simulink model "Group69_Simulink"  (R2021b)
settings: Solver=ode45  StartTime=0.0  StopTime=T  RelTol=1e-12
values from neighbouring files (symbols this model uses):
  A_BN_0 = A_NB_0'    [Group69_Matlab.m]
  m = [0.01 0.05 0.01]'    [Group69_Matlab.m]
  R3H0 = orbit.Re^3*H0    [Group69_Matlab.m]
  w0 = [wx0,wy0,wz0]'    [Group69_Matlab.m]
undefined symbols (not defined in the file or in its folder): gyro, hs, inertia, mag, orbit, r0, rw, sc, t, v0
libraries: matrix_library x8, simulink_extras x6
settings Model: Creator=rocco_larocca  LastModifiedBy=rocco_larocca

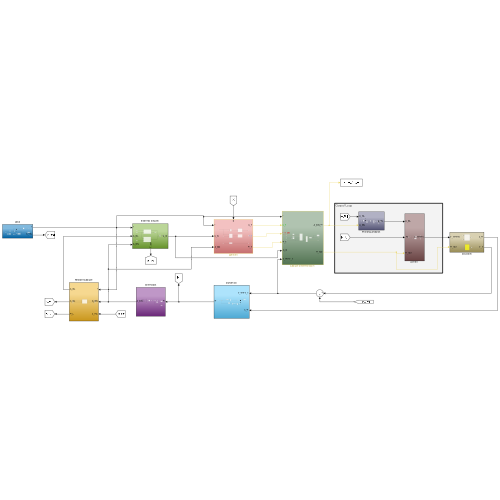
[thumbnail: Simulink's stored preview of the top-level diagram]
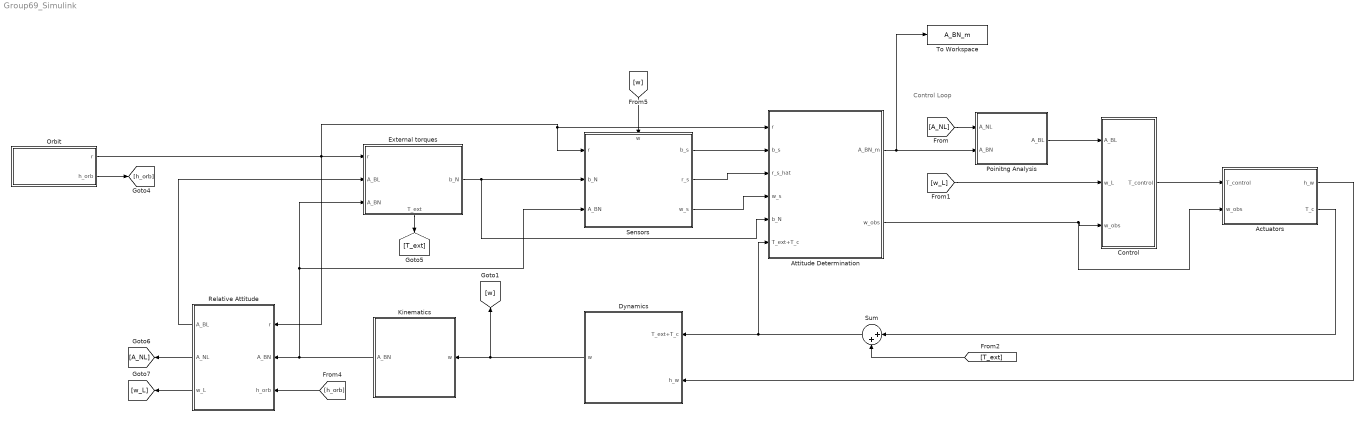
== system Group69_Simulink ==
  note: Control Loop
  Actuators : Subsystem
  "Attitude Determination " : Subsystem
  Control : Subsystem
  Dynamics : Subsystem
  External torques : Subsystem
      settings: PortSchema="{\"entries\":[{\"content\":{\"sides\":[{\"content\":{\"connectorIds\":[\"In1\",\"In2\",\"In3\"]},\"type\":\"ConnectorPlacement.EquallySpacedRectSide\",\"uuid\":\"c5dd5657-11cd-46fc-a813-74747ea81146\"},{\"content\":{\"connectorIds\":[\"Out1\"],\"side\":\"RIGHT\"},\"type\":\"ConnectorPlacement.EquallySpacedRectSide\",\"uuid\":\"ce8cbc86-0401-4f30-83b3-f262a6771dee\"},{\"content\":{\"connectorIds\":[],\"side\":\"TOP\"},\"type\":\"ConnectorPlacement.EquallySpacedRectSide\",\"uuid\":\"54f7f4d9-1155-478d-825b-4623d6763012\"},{\"content\":{\"connectorIds\":[\"Out2\"],\"side\":\"BOTTOM\"},\"type\":\"ConnectorPlacement.EquallySpacedRectSide\",\"uuid\":\"9bbeb954-f49a-41a5-9c63-5058200ec5df\"}]},\"type\":\"ConnectorPlacement.EquallySpacedConnector\",\"uuid\":\"ae160f86-5b24-4f86-a6f1-a9e1b48113ae\"}],\"packageUris\":[\"http://schema.mathworks.com/mf0/Connector/R2020b\"],\"version\":\"1.0\"}"
  Kinematics : Subsystem
  Orbit : Subsystem
  Poinitng Analysis : Subsystem
  Relative Attitude : Subsystem
  Sensors : Subsystem
      settings: PortSchema="{\"entries\":[{\"content\":{\"sides\":[{\"content\":{\"connectorIds\":[\"In1\",\"In2\",\"In3\"]},\"type\":\"ConnectorPlacement.EquallySpacedRectSide\",\"uuid\":\"26d18e7d-7ebd-44fe-966b-e5460611b065\"},{\"content\":{\"connectorIds\":[\"Out1\",\"Out2\",\"Out3\"],\"side\":\"RIGHT\"},\"type\":\"ConnectorPlacement.EquallySpacedRectSide\",\"uuid\":\"31c3f243-0c2a-44fb-92ca-61b97f920180\"},{\"content\":{\"connectorIds\":[\"In4\"],\"side\":\"TOP\"},\"type\":\"ConnectorPlacement.EquallySpacedRectSide\",\"uuid\":\"517f47c7-f5cc-49ce-9a5d-236df56a8d72\"}]},\"type\":\"ConnectorPlacement.EquallySpacedConnector\",\"uuid\":\"aa3704da-9102-4b45-8547-3c2cdec151e6\"}],\"packageUris\":[\"http://schema.mathworks.com/mf0/Connector/R2020b\"],\"version\":\"1.0\"}"
  Sum : Sum  Inputs=|++
  To Workspace : ToWorkspace  VariableName=A_BN_m  SaveFormat=Timeseries  SampleTime=-1
  wires:
  Dynamics/1(w) -> [w], Kinematics/1(w)
  Kinematics/1(A_BN) -> Sensors/3(A_BN), External torques/3(A_BN), Relative Attitude/2(A_BN)
  [h_orb] -> Relative Attitude/3(h_orb)
  Orbit/1(r) -> Relative Attitude/1(r), Sensors/1(r), "Attitude Determination "/1(r), External torques/1(r)
  Orbit/2(h_orb) -> [h_orb]
  Relative Attitude/1(A_BL) -> External torques/2(A_BL)
  External torques/2(T_ext) -> [T_ext]
  External torques/1(b_N) -> "Attitude Determination "/5(" b_N "), Sensors/2(b_N)
  [w] -> Sensors/4(w)
  Sensors/2(r_s) -> "Attitude Determination "/3(r_s_hat)
  Sensors/1(b_s) -> "Attitude Determination "/2(b_s)
  Sensors/3(w_s) -> "Attitude Determination "/4(w_s)
  Relative Attitude/2(A_NL) -> [A_NL]
  Relative Attitude/3(w_L) -> [w_L]
  [T_ext] -> Sum/2
  Actuators/2(T_c) -> Sum/1
  Sum/1 -> "Attitude Determination "/6(T_ext+T_c), Dynamics/1(T_ext+T_c)
  Actuators/1(h_w) -> Dynamics/2(h_w)
  [A_NL] -> Poinitng Analysis/1(A_NL)
  "Attitude Determination "/1(A_BN_m) -> To Workspace/1, Poinitng Analysis/2(A_BN)
  Poinitng Analysis/1(A_BL) -> Control/1(A_BL)
  "Attitude Determination "/2(w_obs) -> Actuators/2(w_obs), Control/3("w_obs ")
  Control/1(T_control) -> Actuators/1(T_control)
  [w_L] -> Control/2(" w_L ")

== system Group69_Simulink/Actuators ==
  T_control : Inport
  w_obs : Inport  Port=2
  Inertia Wheel : Subsystem
      settings: PortSchema="{\"entries\":[{\"content\":{\"sides\":[{\"content\":{\"connectorIds\":[]},\"type\":\"ConnectorPlacement.EquallySpacedRectSide\",\"uuid\":\"666c479f-9627-4b2d-b95f-c868510cc6c0\"},{\"content\":{\"connectorIds\":[],\"side\":\"RIGHT\"},\"type\":\"ConnectorPlacement.EquallySpacedRectSide\",\"uuid\":\"1c954fcd-03c3-4322-8621-3bafaef6b025\"},{\"content\":{\"connectorIds\":[],\"side\":\"TOP\"},\"type\":\"ConnectorPlacement.EquallySpacedRectSide\",\"uuid\":\"948c880d-c243-4d30-bb3c-bd369bf7890c\"},{\"content\":{\"connectorIds\":[\"Out1\"],\"side\":\"BOTTOM\"},\"type\":\"ConnectorPlacement.EquallySpacedRectSide\",\"uuid\":\"e6b921d4-3671-426f-8404-dd4d7604816b\"}]},\"type\":\"ConnectorPlacement.EquallySpacedConnector\",\"uuid\":\"4740817b-bbe6-45b7-9db2-684bb8b90ddd\"}],\"packageUris\":[\"http://schema.mathworks.com/mf0/Connector/R2020b\"],\"version\":\"1.0\"}"
  Reaction Wheels : Subsystem
  h_w : Outport
  T_c : Outport  Port=2
  wires:
  T_control/1 -> Reaction Wheels/1(T_control)
  Reaction Wheels/1(T_c) -> T_c/1
  w_obs/1 -> Reaction Wheels/2(w_obs)
  Inertia Wheel/1(h_w) -> h_w/1

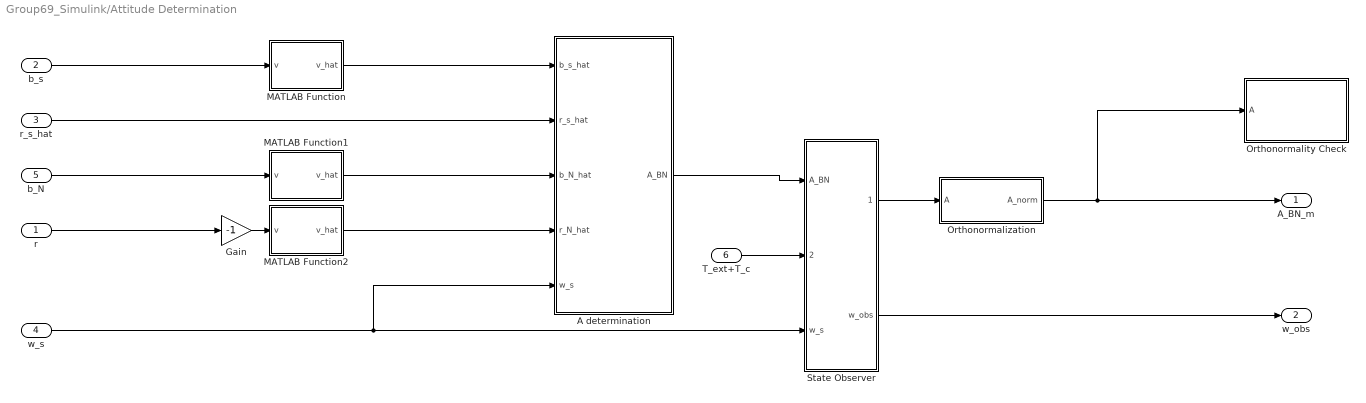
== system Group69_Simulink/Attitude Determination  ==
  r : Inport
  b_s : Inport  Port=2
  r_s_hat : Inport  Port=3
  w_s : Inport  Port=4
  " b_N " : Inport  Port=5
  T_ext+T_c : Inport  Port=6
  A determination : Subsystem
  Gain : Gain  Gain=-1
  MATLAB Function : MATLAB Function  TreatAsAtomicUnit=on
  MATLAB Function1 : MATLAB Function  TreatAsAtomicUnit=on
  MATLAB Function2 : MATLAB Function  TreatAsAtomicUnit=on
  Orthonormality Check : Subsystem
  Orthonormalization : Subsystem
  State Observer : Subsystem
  A_BN_m : Outport
  w_obs : Outport  Port=2
  wires:
  r/1 -> Gain/1
  b_s/1 -> MATLAB Function/1(v)
  Gain/1 -> MATLAB Function2/1(v)
  " b_N "/1 -> MATLAB Function1/1(v)
  r_s_hat/1 -> A determination/2(r_s_hat)
  Orthonormalization/1(A_norm) -> Orthonormality Check/1(A), A_BN_m/1
  w_s/1 -> State Observer/3(w_s), A determination/5(w_s)
  State Observer/1(A_BN_obs) -> Orthonormalization/1(A)
  A determination/1(A_BN) -> State Observer/1(A_BN)
  MATLAB Function/1(v_hat) -> A determination/1(b_s_hat)
  MATLAB Function1/1(v_hat) -> A determination/3(b_N_hat)
  MATLAB Function2/1(v_hat) -> A determination/4(r_N_hat)
  T_ext+T_c/1 -> State Observer/2(T_ext+T_c)
  State Observer/2(w_obs) -> w_obs/1

== system Group69_Simulink/Control ==
  A_BL : Inport
  " w_L " : Inport  Port=2
  "w_obs " : Inport  Port=3
  Clock : Clock
  Detumbling : Subsystem  TreatAsAtomicUnit=on
  If Action Subsystem : Subsystem  TreatAsAtomicUnit=on
  Merge : Merge
  Phase Identification : If  IfExpression=u1<(300)
  T_control : Outport
  wires:
  Phase Identification/2 -> If Action Subsystem/Action
  A_BL/1 -> If Action Subsystem/1(A_BL)
  " w_L "/1 -> If Action Subsystem/2("w_L  ")
  Clock/1 -> Phase Identification/1
  "w_obs "/1 -> Detumbling/1(w_obs), If Action Subsystem/3(w_b)
  Merge/1 -> T_control/1
  Phase Identification/1 -> Detumbling/Action
  Detumbling/1(T_id) -> Merge/1
  If Action Subsystem/1(T_id) -> Merge/2

== system Group69_Simulink/Dynamics ==
  note: adding inertia wheel
  T_ext+T_c : Inport
  h_w : Inport  Port=2
  Cross Product : matrix_library/Cross Product
      settings: SourceProductBaseCode=SL
  Product : Product  Multiplication=Matrix(*)
  Product1 : Product  Multiplication=Matrix(*)
  Sum : Sum  Inputs=+-
  Sum1 : Sum
  inp1 : Constant  Value=sc.I_inv
  inp2 : Constant  Value=sc.I
  int1 : Integrator  InitialCondition=w0
  out1 : ToWorkspace  VariableName=w  SaveFormat=Timeseries  SampleTime=-1
  w : Outport
  wires:
  Sum/1 -> Product1/2
  Product1/1 -> int1/1
  Product/1 -> Sum1/2
  int1/1 -> Cross Product/1, Product/2, out1/1, w/1
  inp1/1 -> Product1/1
  T_ext+T_c/1 -> Sum/1
  inp2/1 -> Product/1
  Sum1/1 -> Cross Product/2
  h_w/1 -> Sum1/1
  Cross Product/1 -> Sum/2

== system Group69_Simulink/External torques ==
  r : Inport
  A_BL : Inport  Port=2
  A_BN : Inport  Port=3
  Gravity Gradient Torque : Subsystem
  Magnetic Torque : Subsystem
  Sum : Sum
  b_N : Outport
  T_ext : Outport  Port=2
  wires:
  A_BL/1 -> Gravity Gradient Torque/2(A_BL)
  r/1 -> Gravity Gradient Torque/1(r), Magnetic Torque/2(r)
  A_BN/1 -> Magnetic Torque/1(A_BN)
  Sum/1 -> T_ext/1
  Magnetic Torque/1(T_magnetic) -> Sum/1
  Magnetic Torque/2(b_N) -> b_N/1
  Gravity Gradient Torque/1(T_gravity) -> Sum/2

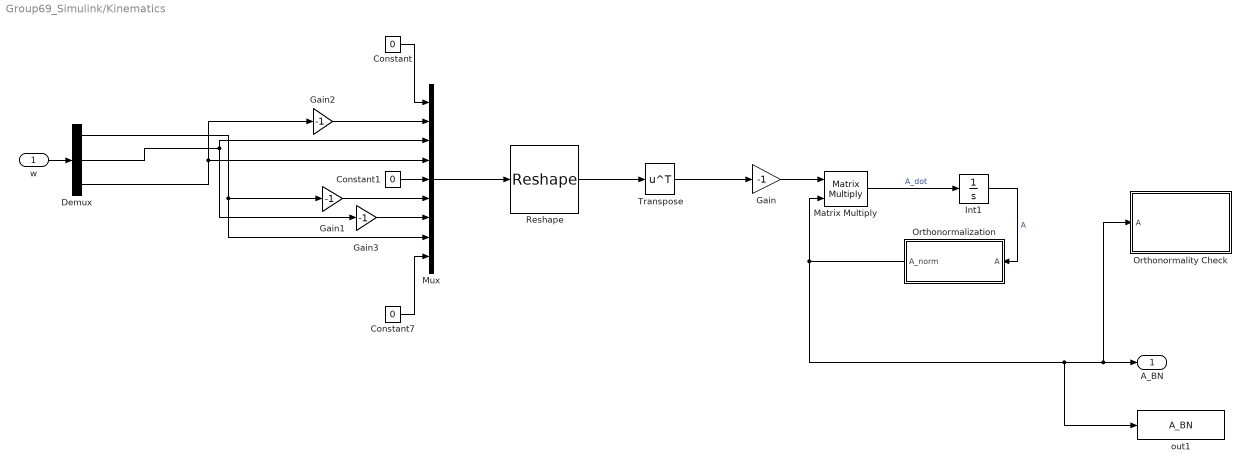
== system Group69_Simulink/Kinematics ==
  w : Inport
  Constant : Constant  Value=0
  Constant1 : Constant  Value=0
  Constant7 : Constant  Value=0
  Demux : Demux  Outputs=3
  Gain{,1..3} (4 alike) : Gain  Gain=-1
  Int1 : Integrator  InitialCondition=A_BN_0
  Matrix Multiply : Product  Multiplication=Matrix(*)
  Mux : Mux  Inputs=9
  Orthonormality Check : Subsystem
  Orthonormalization : Subsystem
  Reshape : Reshape  OutputDimensionality=Customize  OutputDimensions=[3,3]
  Transpose : Math  Operator=transpose  SaturateOnIntegerOverflow=on
  out1 : ToWorkspace  VariableName=A_BN  SaveFormat=Timeseries  SampleTime=-1
  A_BN : Outport
  wires:
  Matrix Multiply/1 -> Int1/1  "A_dot"
  Gain/1 -> Matrix Multiply/1
  Int1/1 -> Orthonormalization/1(A)  "A"
  Orthonormalization/1(A_norm) -> Orthonormality Check/1(A), A_BN/1, out1/1, Matrix Multiply/2
  Constant1/1 -> Mux/5
  Constant/1 -> Mux/1
  Gain1/1 -> Mux/6
  Mux/1 -> Reshape/1
  Gain2/1 -> Mux/2
  Gain3/1 -> Mux/7
  Demux/1 -> Mux/8, Gain1/1
  Constant7/1 -> Mux/9
  w/1 -> Demux/1
  Reshape/1 -> Transpose/1
  Demux/3 -> Mux/4, Gain2/1
  Demux/2 -> Mux/3, Gain3/1
  Transpose/1 -> Gain/1

== system Group69_Simulink/Orbit ==
  Constant : Constant  Value=-3
  Cross Product : matrix_library/Cross Product
      settings: SourceProductBaseCode=SL
  Gain : Gain  Gain=orbit.mu
  Gain1 : Gain  Gain=-1
  MATLAB Function : MATLAB Function  TreatAsAtomicUnit=on
  MatrixMultiply : Product
  Power : Math  Operator=pow  SaturateOnIntegerOverflow=on
  Terminator : Terminator
  To Workspace3 : ToWorkspace  VariableName=r  SaveFormat=Timeseries  SampleTime=-1
  int1 : Integrator  InitialCondition=v0
  int2 : Integrator  InitialCondition=r0
  r : Outport
  h_orb : Outport  Port=2
  wires:
  Gain/1 -> Gain1/1
  int2/1 -> MATLAB Function/1(v), To Workspace3/1, Cross Product/1, r/1, MatrixMultiply/1
  Gain1/1 -> int1/1
  int1/1 -> Cross Product/2, int2/1
  MatrixMultiply/1 -> Gain/1
  Power/1 -> MatrixMultiply/2
  Constant/1 -> Power/2
  Cross Product/1 -> h_orb/1
  MATLAB Function/2(norm_v) -> Power/1
  MATLAB Function/1(v_hat) -> Terminator/1

== system Group69_Simulink/Poinitng Analysis ==
  A_NL : Inport
  A_BN : Inport  Port=2
  Acos : Trigonometry  Operator=acos
  Dot Product : DotProduct  InputSameDT=on  OutDataTypeStr=Inherit: Inherit via internal rule
  MatrixMultiply : Product  Multiplication=Matrix(*)
  MatrixMultiply1 : Product  Multiplication=Matrix(*)
  Nadir Pointing in Body : Constant  Value=[ 1 0 0 ]
  Nadir Pointing in LVLH : Constant  Value=[ 1 0 0 ]
  Radians to Degrees : simulink_extras/Transformations/Radians to Degrees
  Scope : Scope
  To Workspace : ToWorkspace  VariableName=ang_err  SaveFormat=Timeseries  SampleTime=-1
  A_BL : Outport
  wires:
  A_NL/1 -> MatrixMultiply/2
  A_BN/1 -> MatrixMultiply/1
  MatrixMultiply/1 -> MatrixMultiply1/1, A_BL/1
  Nadir Pointing in LVLH/1 -> MatrixMultiply1/2
  MatrixMultiply1/1 -> Dot Product/1
  Nadir Pointing in Body/1 -> Dot Product/2
  Dot Product/1 -> Acos/1
  Acos/1 -> Radians to Degrees/1
  Radians to Degrees/1 -> To Workspace/1, Scope/1

== system Group69_Simulink/Relative Attitude ==
  r : Inport
  A_BN : Inport  Port=2
  h_orb : Inport  Port=3
  moving to LVLH and inertial : Subsystem
  A_BL : Outport
  A_NL : Outport  Port=2
  w_L : Outport  Port=3
  wires:
  h_orb/1 -> moving to LVLH and inertial/3(h_orb)
  moving to LVLH and inertial/1(A_BL) -> A_BL/1
  moving to LVLH and inertial/2(A_NL) -> A_NL/1
  A_BN/1 -> moving to LVLH and inertial/1(A_BN)
  r/1 -> moving to LVLH and inertial/2(r)
  moving to LVLH and inertial/3(w_L) -> w_L/1

== system Group69_Simulink/Sensors ==
  r : Inport
  b_N : Inport  Port=2
  A_BN : Inport  Port=3
  w : Inport  Port=4
  Earth Horizon Sensor : Subsystem
  Field of view check and r to body : Subsystem
  From inertial to body : Product  Multiplication=Matrix(*)
  Gyroscope : Subsystem
  Magnetic Sensor : Subsystem
  b_s : Outport
  r_s : Outport  Port=2
  w_s : Outport  Port=3
  wires:
  A_BN/1 -> Field of view check and r to body/1(A_BN), From inertial to body/1
  r/1 -> Field of view check and r to body/2(r)
  Magnetic Sensor/1(b_S) -> b_s/1
  b_N/1 -> From inertial to body/2
  From inertial to body/1 -> Magnetic Sensor/1(b_B)
  Earth Horizon Sensor/1(r_s) -> r_s/1
  Field of view check and r to body/1(r_B) -> Earth Horizon Sensor/1(r_B)
  w/1 -> Gyroscope/1(w)
  Gyroscope/1(w_s) -> w_s/1

== system Group69_Simulink/Actuators/Inertia Wheel ==
  Clock1 : Clock
  Gain : Gain  Gain=0
  MatrixMultiply : Product  Multiplication=Matrix(*)
  Scope : Scope
  Switch : Switch  Criteria=u2 > Threshold  Threshold=t.detumbling
  inp1 : Constant  Value=inertia.I
  inp2 : Constant  Value=inertia.w
  h_w : Outport
  wires:
  inp1/1 -> MatrixMultiply/1
  Gain/1 -> Switch/3
  Clock1/1 -> Switch/2
  inp2/1 -> MatrixMultiply/2
  MatrixMultiply/1 -> Gain/1, Switch/1
  Switch/1 -> h_w/1, Scope/1

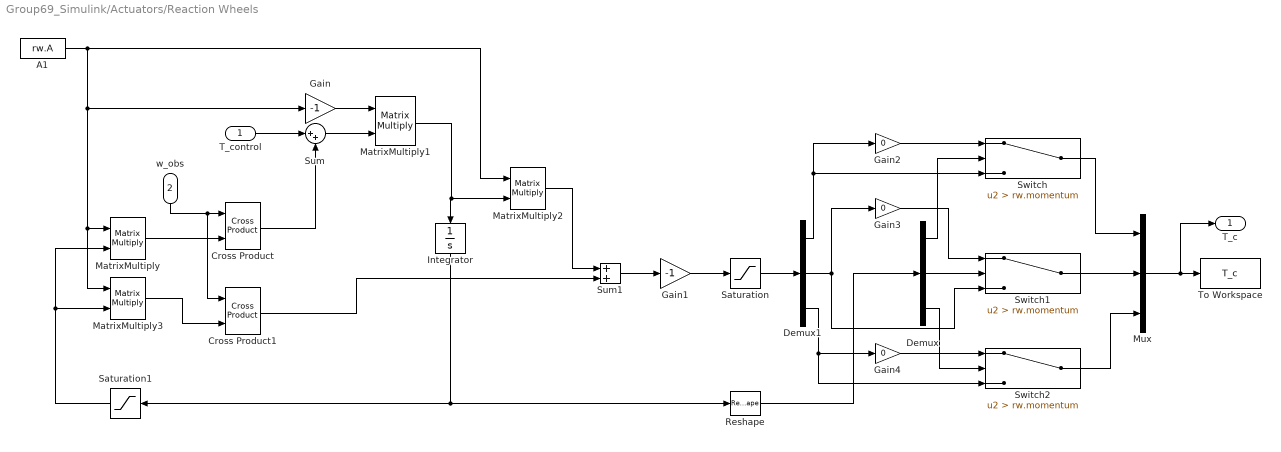
== system Group69_Simulink/Actuators/Reaction Wheels ==
  T_control : Inport
  w_obs : Inport  Port=2
  A1 : Constant  Value=rw.A
  Cross Product : matrix_library/Cross Product
      settings: SourceProductBaseCode=SL
  Cross Product1 : matrix_library/Cross Product
      settings: SourceProductBaseCode=SL
  Demux : Demux  Outputs=3
  Demux1 : Demux  Outputs=3
  Gain : Gain  Gain=-1
  Gain1 : Gain  Gain=-1
  Gain2 : Gain  Gain=0
  Gain3 : Gain  Gain=0
  Gain4 : Gain  Gain=0
  Integrator : Integrator
  MatrixMultiply{,1..3} (4 alike) : Product  Multiplication=Matrix(*)
  Mux : Mux  Inputs=3
  Reshape : Reshape  OutputDimensionality=Column vector (2-D)
  Saturation : Saturate  UpperLimit=rw.maxtorque  LowerLimit=-rw.maxtorque  LinearizeAsGain=off
  Saturation1 : Saturate  UpperLimit=rw.momentum  LowerLimit=-rw.momentum
  Sum : Sum  Inputs=|++
  Sum1 : Sum
  Switch : Switch  Criteria=u2 > Threshold  Threshold=rw.momentum
  Switch1 : Switch  Criteria=u2 > Threshold  Threshold=rw.momentum
  Switch2 : Switch  Criteria=u2 > Threshold  Threshold=rw.momentum
  To Workspace : ToWorkspace  VariableName=T_c  SaveFormat=Timeseries  SampleTime=-1
  T_c : Outport
  wires:
  w_obs/1 -> Cross Product1/1, Cross Product/1
  MatrixMultiply1/1 -> Integrator/1, MatrixMultiply2/2
  Saturation1/1 -> MatrixMultiply/2, MatrixMultiply3/2
  Demux1/1 -> Switch/3, Gain2/1
  Demux1/2 -> Switch1/3, Gain3/1
  Mux/1 -> To Workspace/1, T_c/1
  MatrixMultiply/1 -> Cross Product/2
  T_control/1 -> Sum/1
  Cross Product1/1 -> Sum1/2
  Cross Product/1 -> Sum/2
  Sum/1 -> MatrixMultiply1/2
  Gain/1 -> MatrixMultiply1/1
  MatrixMultiply2/1 -> Sum1/1
  Sum1/1 -> Gain1/1
  Gain1/1 -> Saturation/1
  MatrixMultiply3/1 -> Cross Product1/2
  Demux/2 -> Switch1/2
  Demux/3 -> Switch2/2
  Switch1/1 -> Mux/2
  Gain3/1 -> Switch1/1
  Gain2/1 -> Switch/1
  Switch/1 -> Mux/1
  Demux/1 -> Switch/2
  Gain4/1 -> Switch2/1
  Switch2/1 -> Mux/3
  Reshape/1 -> Demux/1
  Saturation/1 -> Demux1/1
  Demux1/3 -> Switch2/3, Gain4/1
  Integrator/1 -> Saturation1/1, Reshape/1
  A1/1 -> MatrixMultiply2/1, Gain/1, MatrixMultiply3/1, MatrixMultiply/1

== system Group69_Simulink/Attitude Determination /A determination ==
  b_s_hat : Inport
  r_s_hat : Inport  Port=2
  b_N_hat : Inport  Port=3
  r_N_hat : Inport  Port=4
  w_s : Inport  Port=5
  A_det : MATLAB Function  TreatAsAtomicUnit=on
  Reshape{,2..3,5} (4 alike) : Reshape  OutputDimensionality=Column vector (2-D)
  Subsystem : Subsystem
  A_BN : Outport
  wires:
  b_s_hat/1 -> Reshape/1
  r_s_hat/1 -> Reshape2/1
  b_N_hat/1 -> Reshape3/1
  r_N_hat/1 -> Reshape5/1
  Reshape/1 -> A_det/1(b_s_hat)
  Reshape2/1 -> A_det/2(r_s_hat)
  Reshape3/1 -> A_det/3(b_N_hat)
  Reshape5/1 -> A_det/4(r_N_hat)
  w_s/1 -> A_det/5(wb_sens)
  Subsystem/1(A_BN) -> A_BN/1
  Subsystem/2(A_prev) -> A_det/6(A_prev)
  A_det/2(c) -> Subsystem/2(c)
  A_det/1(A) -> Subsystem/1(A)
  A_det/3(A_dot) -> Subsystem/3(A_dot)

== system Group69_Simulink/Attitude Determination /Orthonormality Check ==
  A : Inport
  Determinant : Subsystem  Commented=on
  MATLAB Function : MATLAB Function  TreatAsAtomicUnit=on
  Scope : Scope
  wires:
  A/1 -> MATLAB Function/1(A)
  MATLAB Function/1(detA) -> Scope/1

== system Group69_Simulink/Attitude Determination /Orthonormalization ==
  A : Inport
  Gain : Gain  Gain=1.5
  Gain1 : Gain  Gain=0.5
  Matrix Multiply : Product  Multiplication=Matrix(*)
  Matrix Multiply1 : Product  Multiplication=Matrix(*)
  Sum : Sum  Inputs=+-
  Transpose : Math  Operator=transpose  SaturateOnIntegerOverflow=on
  A_norm : Outport
  wires:
  Gain/1 -> Sum/1
  Transpose/1 -> Matrix Multiply/2
  A/1 -> Transpose/1, Gain1/1, Matrix Multiply/1, Gain/1
  Matrix Multiply1/1 -> Sum/2
  Sum/1 -> A_norm/1
  Matrix Multiply/1 -> Matrix Multiply1/1
  Gain1/1 -> Matrix Multiply1/2

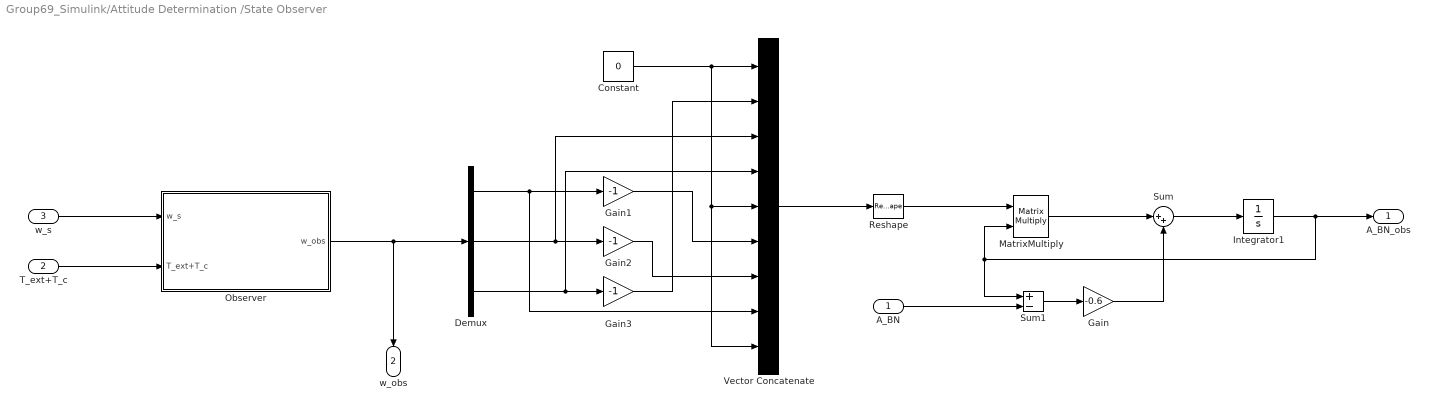
== system Group69_Simulink/Attitude Determination /State Observer ==
  A_BN : Inport
  T_ext+T_c : Inport  Port=2
  w_s : Inport  Port=3
  Constant : Constant  Value=0
  Demux : Demux  Outputs=3
  Gain : Gain  Gain=-0.6
  Gain1 : Gain  Gain=-1
  Gain2 : Gain  Gain=-1
  Gain3 : Gain  Gain=-1
  Integrator1 : Integrator  InitialCondition=A_BN_0
  MatrixMultiply : Product  Multiplication=Matrix(*)
  Observer : Subsystem
  Reshape : Reshape  OutputDimensionality=Customize  OutputDimensions=[3,3]
  Sum : Sum  Inputs=|++
  Sum1 : Sum  Inputs=+-
  Vector Concatenate : Concatenate  NumInputs=9
  A_BN_obs : Outport
  w_obs : Outport  Port=2
  wires:
  MatrixMultiply/1 -> Sum/1
  Sum1/1 -> Gain/1
  Integrator1/1 -> A_BN_obs/1, MatrixMultiply/2, Sum1/1
  A_BN/1 -> Sum1/2
  Gain/1 -> Sum/2
  Reshape/1 -> MatrixMultiply/1
  Sum/1 -> Integrator1/1
  Demux/1 -> Vector Concatenate/8, Gain1/1
  Demux/3 -> Gain3/1, Vector Concatenate/4
  Gain1/1 -> Vector Concatenate/6
  Constant/1 -> Vector Concatenate/1, Vector Concatenate/9, Vector Concatenate/5
  Demux/2 -> Vector Concatenate/3, Gain2/1
  Gain3/1 -> Vector Concatenate/2
  Vector Concatenate/1 -> Reshape/1
  Gain2/1 -> Vector Concatenate/7
  T_ext+T_c/1 -> Observer/2(T_ext+T_c)
  w_s/1 -> Observer/1(w_s)
  Observer/1(w_obs) -> w_obs/1, Demux/1

== system Group69_Simulink/Control/Detumbling ==
  w_obs : Inport
  Action Port : ActionPort  ActionPortLabel=if(u1<(300))
  1 : Gain  Gain=-1e-3
  2 : Gain  Gain=-1e-3
  3 : Gain  Gain=-1e-3
  Demux : Demux  Outputs=3
  Mux2 : Mux  Inputs=3
  T_id : Outport
  wires:
  Demux/1 -> 2/1
  2/1 -> Mux2/1
  3/1 -> Mux2/3
  Demux/2 -> 1/1
  Demux/3 -> 3/1
  1/1 -> Mux2/2
  w_obs/1 -> Demux/1
  Mux2/1 -> T_id/1

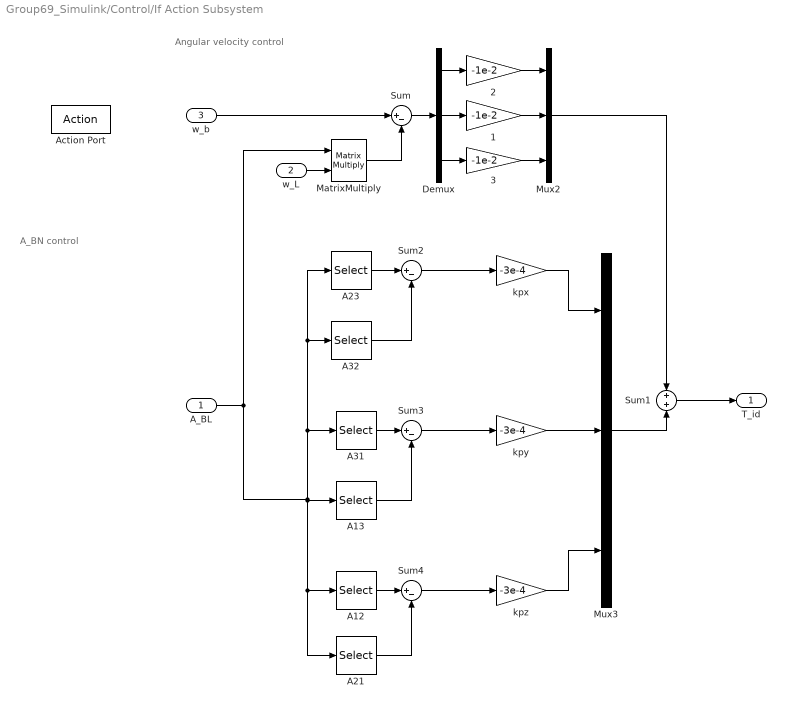
== system Group69_Simulink/Control/If Action Subsystem ==
  note: Angular velocity control
  note: A_BN control
  A_BL : Inport
  "w_L  " : Inport  Port=2
  w_b : Inport  Port=3
  Action Port : ActionPort  ActionPortLabel=else
  1 : Gain  Gain=-1e-2
  2 : Gain  Gain=-1e-2
  3 : Gain  Gain=-1e-2
  A12 : Selector  NumberOfDimensions=2  InputPortWidth=3  IndexOptions=Index vector (dialog),Index vector (dialog)  Indices=1,2  OutputSizes=1,1
  A13 : Selector  NumberOfDimensions=2  InputPortWidth=3  IndexOptions=Index vector (dialog),Index vector (dialog)  Indices=1,3  OutputSizes=1,1
  A21 : Selector  NumberOfDimensions=2  InputPortWidth=3  IndexOptions=Index vector (dialog),Index vector (dialog)  Indices=2,1  OutputSizes=1,1
  A23 : Selector  NumberOfDimensions=2  InputPortWidth=3  IndexOptions=Index vector (dialog),Index vector (dialog)  Indices=2,3  OutputSizes=1,1
  A31 : Selector  NumberOfDimensions=2  InputPortWidth=3  IndexOptions=Index vector (dialog),Index vector (dialog)  Indices=3,1  OutputSizes=1,1
  A32 : Selector  NumberOfDimensions=2  InputPortWidth=3  IndexOptions=Index vector (dialog),Index vector (dialog)  Indices=3,2  OutputSizes=1,1
  Demux : Demux  Outputs=3
  MatrixMultiply : Product  Multiplication=Matrix(*)
  Mux2 : Mux  Inputs=3
  Mux3 : Mux  Inputs=3
  Sum{,2..4} (4 alike) : Sum  Inputs=|+-
  Sum1 : Sum  Inputs=+|+
  kpx : Gain  Gain=-3e-4
  kpy : Gain  Gain=-3e-4
  kpz : Gain  Gain=-3e-4
  T_id : Outport
  wires:
  MatrixMultiply/1 -> Sum/2
  3/1 -> Mux2/3
  1/1 -> Mux2/2
  Demux/1 -> 2/1
  Demux/3 -> 3/1
  w_b/1 -> Sum/1
  Sum/1 -> Demux/1
  2/1 -> Mux2/1
  Demux/2 -> 1/1
  "w_L  "/1 -> MatrixMultiply/2
  Sum1/1 -> T_id/1
  kpx/1 -> Mux3/1
  kpy/1 -> Mux3/2
  kpz/1 -> Mux3/3
  A_BL/1 -> A13/1, A21/1, A12/1, A23/1, A32/1, A31/1, MatrixMultiply/1
  A23/1 -> Sum2/1
  A32/1 -> Sum2/2
  A31/1 -> Sum3/1
  A13/1 -> Sum3/2
  A12/1 -> Sum4/1
  A21/1 -> Sum4/2
  Sum2/1 -> kpx/1
  Sum3/1 -> kpy/1
  Sum4/1 -> kpz/1
  Mux3/1 -> Sum1/2
  Mux2/1 -> Sum1/1

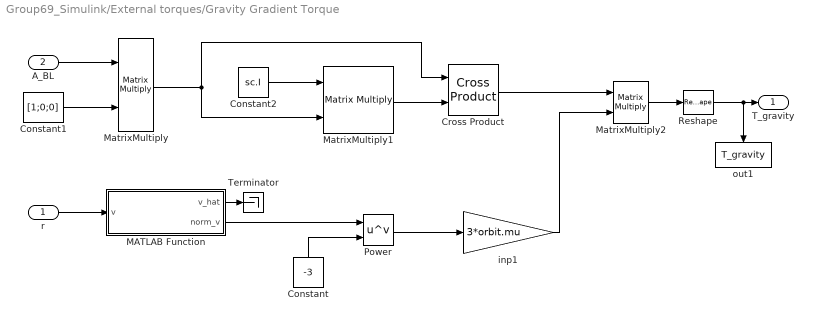
== system Group69_Simulink/External torques/Gravity Gradient Torque ==
  r : Inport
  A_BL : Inport  Port=2
  Constant : Constant  Value=-3
  Constant1 : Constant  Value=[1;0;0]  VectorParams1D=off
  Constant2 : Constant  Value=sc.I  VectorParams1D=off
  Cross Product : matrix_library/Cross Product
      settings: SourceProductBaseCode=SL
  MATLAB Function : MATLAB Function  TreatAsAtomicUnit=on
  MatrixMultiply : Product  Multiplication=Matrix(*)
  MatrixMultiply1 : Product  Multiplication=Matrix(*)
  MatrixMultiply2 : Product  Multiplication=Matrix(*)
  Power : Math  Operator=pow  SaturateOnIntegerOverflow=on
  Reshape : Reshape  OutputDimensionality=Column vector (2-D)
  Terminator : Terminator
  inp1 : Gain  Gain=3*orbit.mu
  out1 : ToWorkspace  VariableName=T_gravity  SaveFormat=Timeseries  SampleTime=-1
  T_gravity : Outport
  wires:
  r/1 -> MATLAB Function/1(v)
  MATLAB Function/2(norm_v) -> Power/1
  Constant/1 -> Power/2
  Power/1 -> inp1/1
  A_BL/1 -> MatrixMultiply/1
  Constant1/1 -> MatrixMultiply/2
  MatrixMultiply/1 -> Cross Product/1, MatrixMultiply1/2
  Constant2/1 -> MatrixMultiply1/1
  MatrixMultiply1/1 -> Cross Product/2
  inp1/1 -> MatrixMultiply2/2
  Cross Product/1 -> MatrixMultiply2/1
  MatrixMultiply2/1 -> Reshape/1
  Reshape/1 -> out1/1, T_gravity/1
  MATLAB Function/1(v_hat) -> Terminator/1

== system Group69_Simulink/External torques/Magnetic Torque ==
  A_BN : Inport
  r : Inport  Port=2
  Clock : Clock
  Cross Product : matrix_library/Cross Product
      settings: SourceProductBaseCode=SL
  MatrixMultiply : Product  Multiplication=Matrix(*)
  Reshape : Reshape  OutputDimensionality=Column vector (2-D)
  inp1 : Constant  Value=m
  mag_field in inertial : Subsystem
  out1 : ToWorkspace  VariableName=T_magnetic  SaveFormat=Timeseries  SampleTime=-1
  T_magnetic : Outport
  b_N : Outport  Port=2
  wires:
  r/1 -> mag_field in inertial/1(r)
  Clock/1 -> mag_field in inertial/2(t)
  mag_field in inertial/1(b_N) -> MatrixMultiply/2, b_N/1
  A_BN/1 -> MatrixMultiply/1
  MatrixMultiply/1 -> Cross Product/2
  inp1/1 -> Cross Product/1
  Cross Product/1 -> Reshape/1
  Reshape/1 -> T_magnetic/1, out1/1

== system Group69_Simulink/Kinematics/Orthonormality Check ==
  A : Inport
  Determinant : Subsystem  Commented=on
  MATLAB Function : MATLAB Function  TreatAsAtomicUnit=on
  Scope : Scope
  wires:
  A/1 -> MATLAB Function/1(A)
  MATLAB Function/1(detA) -> Scope/1

== system Group69_Simulink/Kinematics/Orthonormalization ==
  A : Inport
  Gain : Gain  Gain=1.5
  Gain1 : Gain  Gain=0.5
  Matrix Multiply : Product  Multiplication=Matrix(*)
  Matrix Multiply1 : Product  Multiplication=Matrix(*)
  Sum : Sum  Inputs=+-
  Transpose : Math  Operator=transpose  SaturateOnIntegerOverflow=on
  A_norm : Outport
  wires:
  Gain/1 -> Sum/1
  Transpose/1 -> Matrix Multiply/2
  A/1 -> Transpose/1, Gain1/1, Matrix Multiply/1, Gain/1
  Matrix Multiply1/1 -> Sum/2
  Sum/1 -> A_norm/1
  Matrix Multiply/1 -> Matrix Multiply1/1
  Gain1/1 -> Matrix Multiply1/2

== system Group69_Simulink/Relative Attitude/moving to LVLH and inertial ==
  A_BN : Inport
  r : Inport  Port=2
  h_orb : Inport  Port=3
  DCM from L to N : Subsystem
  MatrixMultiply : Product  Multiplication=Matrix(*)
  Subsystem : Subsystem
  out1 : ToWorkspace  VariableName=A_NL  SaveFormat=Timeseries  SampleTime=-1
  A_BL : Outport
  A_NL : Outport  Port=2
  w_L : Outport  Port=3
  wires:
  DCM from L to N/1(A_NL) -> out1/1, A_NL/1, MatrixMultiply/2
  MatrixMultiply/1 -> A_BL/1
  A_BN/1 -> MatrixMultiply/1
  h_orb/1 -> Subsystem/2(h_orb), DCM from L to N/2(h_orb)
  r/1 -> Subsystem/1(r), DCM from L to N/1(r)
  Subsystem/1(w_L) -> w_L/1

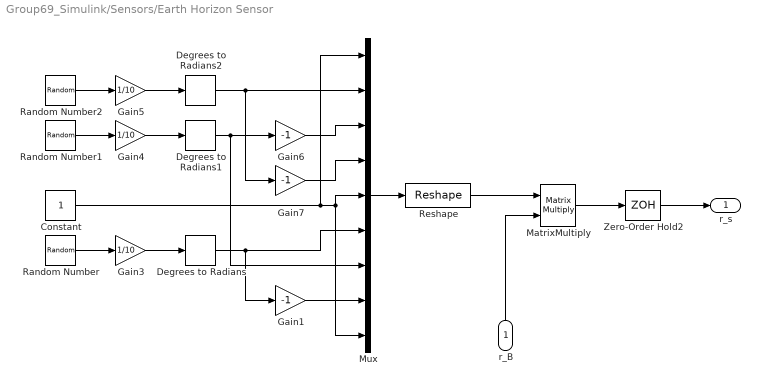
== system Group69_Simulink/Sensors/Earth Horizon Sensor ==
  r_B : Inport
  Constant : Constant
  Degrees to Radians : simulink_extras/Transformations/Degrees to Radians
  Degrees to Radians1 : simulink_extras/Transformations/Degrees to Radians
  Degrees to Radians2 : simulink_extras/Transformations/Degrees to Radians
  Gain1 : Gain  Gain=-1
  Gain3 : Gain  Gain=1/10
  Gain4 : Gain  Gain=1/10
  Gain5 : Gain  Gain=1/10
  Gain6 : Gain  Gain=-1
  Gain7 : Gain  Gain=-1
  MatrixMultiply : Product  Multiplication=Matrix(*)
  Mux : Mux  Inputs=9
  Random Number : RandomNumber  Variance=hs.accuracy^2  Seed=randi([0 400],1,1)  SampleTime=hs.sampling_time
  Random Number1 : RandomNumber  Variance=hs.accuracy^2  Seed=randi([0 400],1,1)  SampleTime=hs.sampling_time
  Random Number2 : RandomNumber  Variance=hs.accuracy^2  Seed=randi([0 400],1,1)  SampleTime=hs.sampling_time
  Reshape : Reshape  OutputDimensionality=Customize  OutputDimensions=[3,3]
  Zero-Order Hold2 : ZeroOrderHold  SampleTime=hs.sampling_time
  r_s : Outport
  wires:
  MatrixMultiply/1 -> Zero-Order Hold2/1
  r_B/1 -> MatrixMultiply/2
  Zero-Order Hold2/1 -> r_s/1
  Gain6/1 -> Mux/3
  Gain1/1 -> Mux/8
  Gain4/1 -> Degrees to Radians1/1
  Degrees to Radians1/1 -> Mux/7, Gain6/1
  Constant/1 -> Mux/9, Mux/5, Mux/1
  Random Number2/1 -> Gain5/1
  Mux/1 -> Reshape/1
  Degrees to Radians2/1 -> Mux/2, Gain7/1
  Random Number1/1 -> Gain4/1
  Gain5/1 -> Degrees to Radians2/1
  Gain3/1 -> Degrees to Radians/1
  Gain7/1 -> Mux/4
  Random Number/1 -> Gain3/1
  Degrees to Radians/1 -> Mux/6, Gain1/1
  Reshape/1 -> MatrixMultiply/1

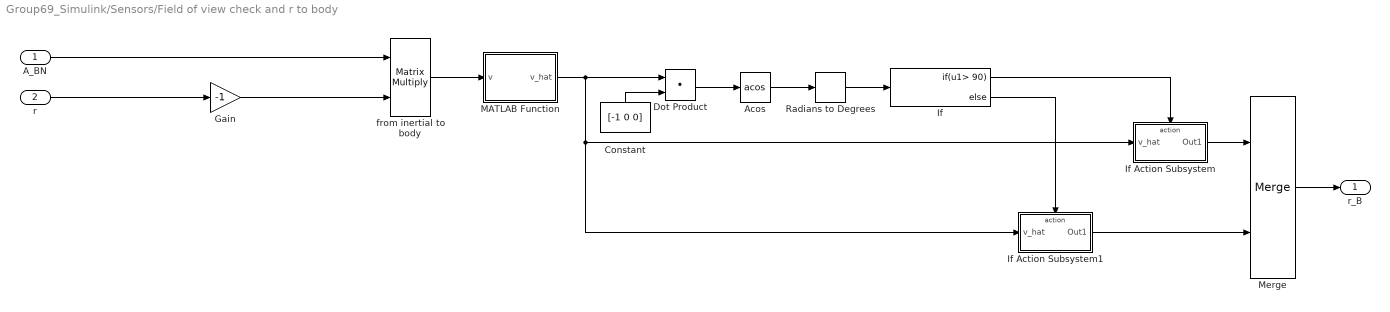
== system Group69_Simulink/Sensors/Field of view check and r to body ==
  A_BN : Inport
  r : Inport  Port=2
  Acos : Trigonometry  Operator=acos
  Constant : Constant  Value=[-1 0 0]
  Dot Product : DotProduct  InputSameDT=on  OutDataTypeStr=Inherit: Inherit via internal rule
  Gain : Gain  Gain=-1
  If : If  IfExpression=u1> 90
  If Action Subsystem : Subsystem  TreatAsAtomicUnit=on
  If Action Subsystem1 : Subsystem  TreatAsAtomicUnit=on
  MATLAB Function : MATLAB Function  TreatAsAtomicUnit=on
  Merge : Merge
  Radians to Degrees : simulink_extras/Transformations/Radians to Degrees
  from inertial to body : Product  Multiplication=Matrix(*)
  r_B : Outport
  wires:
  from inertial to body/1 -> MATLAB Function/1(v)
  MATLAB Function/1(v_hat) -> Dot Product/1, If Action Subsystem1/1(v_hat), If Action Subsystem/1(v_hat)
  Radians to Degrees/1 -> If/1
  Merge/1 -> r_B/1
  If Action Subsystem/1(Out1) -> Merge/1
  If Action Subsystem1/1(Out1) -> Merge/2
  If/2 -> If Action Subsystem1/Action
  If/1 -> If Action Subsystem/Action
  Constant/1 -> Dot Product/2
  Acos/1 -> Radians to Degrees/1
  Dot Product/1 -> Acos/1
  A_BN/1 -> from inertial to body/1
  Gain/1 -> from inertial to body/2
  r/1 -> Gain/1

== system Group69_Simulink/Sensors/Gyroscope ==
  w : Inport
  Add : Sum  Inputs=+++
  Integrator : Integrator
  Random Number : RandomNumber  Variance=(gyro.ARW/sqrt(3600)*pi/180*sqrt(gyro.sampling_time))^2  SampleTime=gyro.sampling_time  VectorParams1D=off
  Random Number1 : RandomNumber  Variance=(gyro.bias/3600*pi/180*sqrt(gyro.sampling_time))^2  SampleTime=gyro.sampling_time
  Zero-Order Hold : ZeroOrderHold  SampleTime=gyro.sampling_time
  w_s : Outport
  wires:
  Add/1 -> Zero-Order Hold/1
  Zero-Order Hold/1 -> w_s/1
  Random Number1/1 -> Integrator/1
  w/1 -> Add/1
  Random Number/1 -> Add/2
  Integrator/1 -> Add/3

== system Group69_Simulink/Sensors/Magnetic Sensor ==
  b_B : Inport
  MatrixMultiply : Product  Multiplication=Matrix(*)
  Saturation : Saturate  UpperLimit=mag.saturation  LowerLimit=-mag.saturation
  Sum : Sum
  Zero-Order Hold1 : ZeroOrderHold  SampleTime=mag.sampling_time
  inp1 : Constant  Value=mag.A_error
  inp2 : Constant  Value=mag.noise
  b_S : Outport
  wires:
  Sum/1 -> MatrixMultiply/2
  inp2/1 -> Sum/1
  inp1/1 -> MatrixMultiply/1
  MatrixMultiply/1 -> Saturation/1
  Saturation/1 -> Zero-Order Hold1/1
  b_B/1 -> Sum/2
  Zero-Order Hold1/1 -> b_S/1

== system Group69_Simulink/Attitude Determination /A determination/Subsystem ==
  A : Inport
  c : Inport  Port=2
  A_dot : Inport  Port=3
  Constant1 : Constant  Value=2
  Equal : RelationalOperator  Operator===  OutDataTypeStr=boolean  RndMeth=Simplest
  If : If  IfExpression=u1 == 2
  If Action Subsystem : Subsystem  TreatAsAtomicUnit=on
  If Action Subsystem1 : Subsystem  TreatAsAtomicUnit=on
  Integrator : Integrator  ExternalReset=either  InitialConditionSource=external  InitialCondition=eye(3)
  Merge : Merge
  delay1 : UnitDelay  InitialCondition=A_BN_0  SampleTime=-1  HasFrameUpgradeWarning=on
  A_BN : Outport
  A_prev : Outport  Port=2
  wires:
  delay1/1 -> A_prev/1, Integrator/3
  Merge/1 -> delay1/1, A_BN/1
  c/1 -> If/1, Equal/1
  If Action Subsystem1/1(Out1) -> Merge/1
  Equal/1 -> Integrator/2
  If Action Subsystem/1(Out1) -> Merge/2
  Constant1/1 -> Equal/2
  If/1 -> If Action Subsystem/Action
  If/2 -> If Action Subsystem1/Action
  Integrator/1 -> If Action Subsystem/1(In1)
  A/1 -> If Action Subsystem1/1(A)
  A_dot/1 -> Integrator/1

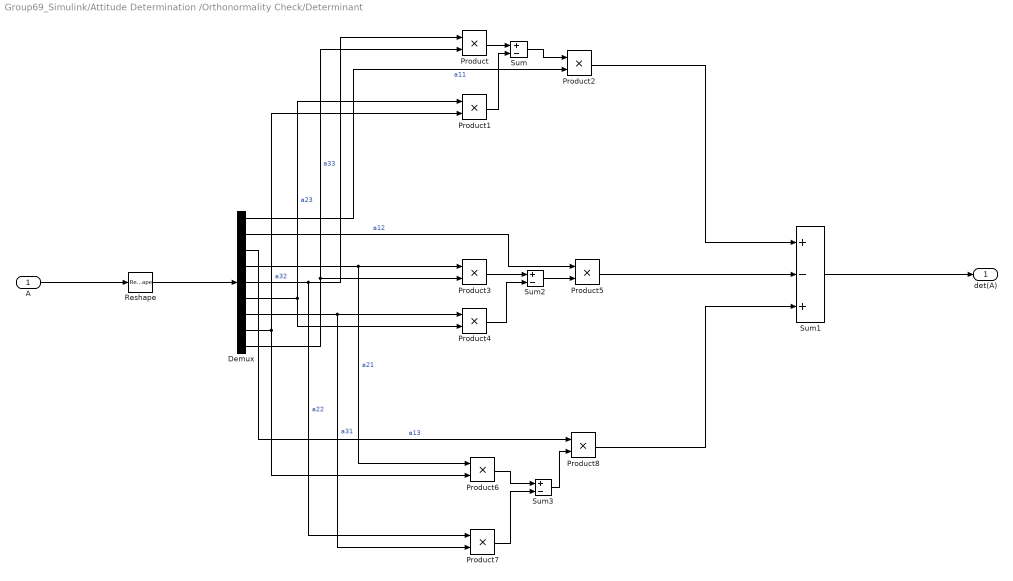
== system Group69_Simulink/Attitude Determination /Orthonormality Check/Determinant ==
  A : Inport
  Demux : Demux  Outputs=9
  Product{,1..8} (9 alike) : Product
  Reshape : Reshape  OutputDimensionality=Customize  OutputDimensions=[9,1]
  Sum : Sum  Inputs=+-
  Sum1 : Sum  Inputs=+-+
  Sum2 : Sum  Inputs=+-
  Sum3 : Sum  Inputs=+-
  det(A) : Outport
  wires:
  Product/1 -> Sum/1
  Demux/5 -> Product7/1, Product/1  "a22"
  Demux/9 -> Product3/2, Product/2  "a33"
  Demux/6 -> Product1/1, Product4/2  "a23"
  Demux/8 -> Product1/2, Product6/2  "a32"
  Product1/1 -> Sum/2
  Demux/1 -> Product2/2  "a11"
  Sum/1 -> Product2/1
  Demux/4 -> Product6/1, Product3/1  "a21"
  Demux/7 -> Product7/2, Product4/1  "a31"
  Product3/1 -> Sum2/1
  Product4/1 -> Sum2/2
  Sum2/1 -> Product5/2
  Demux/2 -> Product5/1  "a12"
  Product2/1 -> Sum1/1
  Product5/1 -> Sum1/2
  Product6/1 -> Sum3/1
  Product7/1 -> Sum3/2
  Sum3/1 -> Product8/2
  Demux/3 -> Product8/1  "a13"
  Product8/1 -> Sum1/3
  Sum1/1 -> det(A)/1
  Reshape/1 -> Demux/1
  A/1 -> Reshape/1

== system Group69_Simulink/Attitude Determination /State Observer/Observer ==
  w_s : Inport
  T_ext+T_c : Inport  Port=2
  Cross Product : matrix_library/Cross Product
      settings: SourceProductBaseCode=SL
  Gain : Gain  Gain=sc.I_inv  Multiplication=Matrix(K*u) (u vector)
  Gain1 : Gain  Gain=sc.I  Multiplication=Matrix(K*u) (u vector)
  Gain2 : Gain  Gain=-0.5
  Integrator1 : Integrator  InitialConditionSource=external
  Sum : Sum  Inputs=+++
  Sum1 : Sum  Inputs=+-
  w_obs : Outport
  wires:
  Gain/1 -> Integrator1/1
  w_s/1 -> Sum1/2, Integrator1/2
  T_ext+T_c/1 -> Sum/2
  Gain2/1 -> Sum/3
  Sum/1 -> Gain/1
  Cross Product/1 -> Sum/1
  Sum1/1 -> Gain2/1
  Gain1/1 -> Cross Product/1
  Integrator1/1 -> Cross Product/2, Sum1/1, Gain1/1, w_obs/1

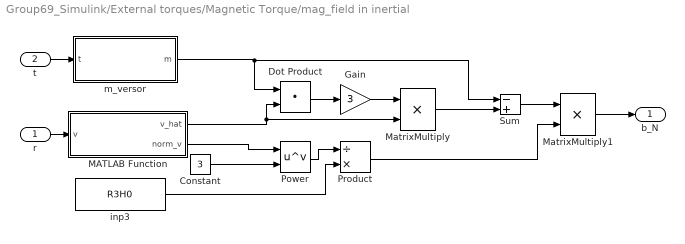
== system Group69_Simulink/External torques/Magnetic Torque/mag_field in inertial ==
  r : Inport
  t : Inport  Port=2
  Constant : Constant  Value=3
  Dot Product : DotProduct  InputSameDT=on  OutDataTypeStr=Inherit: Inherit via internal rule
  Gain : Gain  Gain=3
  MATLAB Function : MATLAB Function  TreatAsAtomicUnit=on
  MatrixMultiply : Product
  MatrixMultiply1 : Product
  Power : Math  Operator=pow  SaturateOnIntegerOverflow=on
  Product : Product  Inputs=/*
  Sum : Sum  Inputs=-+
  inp3 : Constant  Value=R3H0
  m_versor : Subsystem
  b_N : Outport
  wires:
  r/1 -> MATLAB Function/1(v)
  t/1 -> m_versor/1(t)
  MATLAB Function/2(norm_v) -> Power/1
  Constant/1 -> Power/2
  Power/1 -> Product/1
  inp3/1 -> Product/2
  m_versor/1(m) -> Sum/1, Dot Product/1
  MATLAB Function/1(v_hat) -> MatrixMultiply/2, Dot Product/2
  Sum/1 -> MatrixMultiply1/1
  Product/1 -> MatrixMultiply1/2
  MatrixMultiply1/1 -> b_N/1
  Dot Product/1 -> Gain/1
  Gain/1 -> MatrixMultiply/1
  MatrixMultiply/1 -> Sum/2

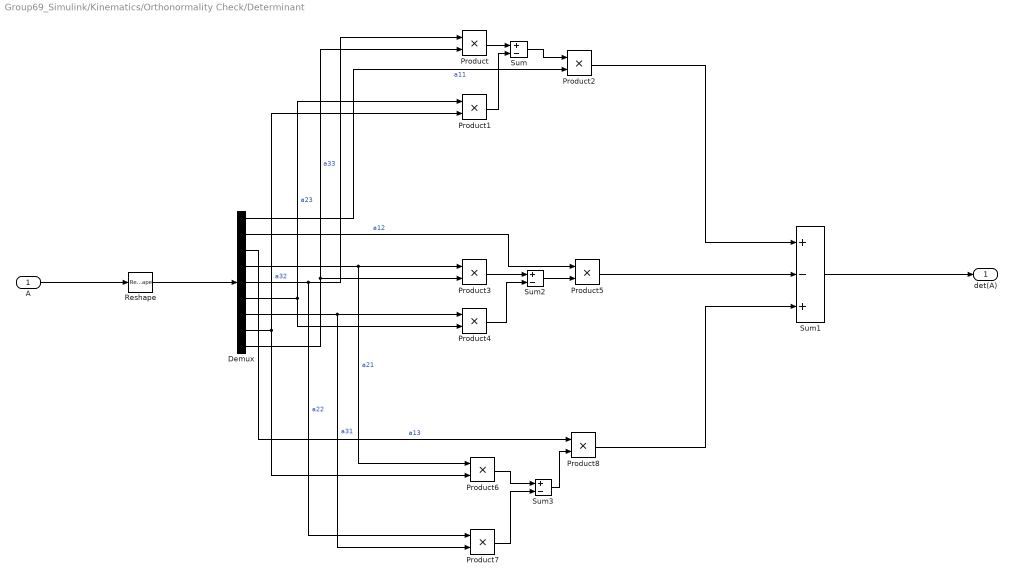
== system Group69_Simulink/Kinematics/Orthonormality Check/Determinant ==
  A : Inport
  Demux : Demux  Outputs=9
  Product{,1..8} (9 alike) : Product
  Reshape : Reshape  OutputDimensionality=Customize  OutputDimensions=[9,1]
  Sum : Sum  Inputs=+-
  Sum1 : Sum  Inputs=+-+
  Sum2 : Sum  Inputs=+-
  Sum3 : Sum  Inputs=+-
  det(A) : Outport
  wires:
  Product/1 -> Sum/1
  Demux/5 -> Product7/1, Product/1  "a22"
  Demux/9 -> Product3/2, Product/2  "a33"
  Demux/6 -> Product1/1, Product4/2  "a23"
  Demux/8 -> Product1/2, Product6/2  "a32"
  Product1/1 -> Sum/2
  Demux/1 -> Product2/2  "a11"
  Sum/1 -> Product2/1
  Demux/4 -> Product6/1, Product3/1  "a21"
  Demux/7 -> Product7/2, Product4/1  "a31"
  Product3/1 -> Sum2/1
  Product4/1 -> Sum2/2
  Sum2/1 -> Product5/2
  Demux/2 -> Product5/1  "a12"
  Product2/1 -> Sum1/1
  Product5/1 -> Sum1/2
  Product6/1 -> Sum3/1
  Product7/1 -> Sum3/2
  Sum3/1 -> Product8/2
  Demux/3 -> Product8/1  "a13"
  Product8/1 -> Sum1/3
  Sum1/1 -> det(A)/1
  Reshape/1 -> Demux/1
  A/1 -> Reshape/1

== system Group69_Simulink/Relative Attitude/moving to LVLH and inertial/DCM from L to N ==
  r : Inport
  h_orb : Inport  Port=2
  Cross Product : matrix_library/Cross Product
      settings: SourceProductBaseCode=SL
  Gain : Gain  Gain=-1
  MATLAB Function : MATLAB Function  TreatAsAtomicUnit=on
  MATLAB Function1 : MATLAB Function  TreatAsAtomicUnit=on
  Mux : Mux  Inputs=3
  Reshape : Reshape  OutputDimensionality=Customize  OutputDimensions=[3,3]
  A_NL : Outport
  wires:
  r/1 -> MATLAB Function/1(v)
  h_orb/1 -> MATLAB Function1/1(v)
  MATLAB Function/1(v_hat) -> Cross Product/1, Mux/1
  MATLAB Function1/1(v_hat) -> Cross Product/2, Mux/3
  Mux/1 -> Reshape/1
  Cross Product/1 -> Gain/1
  Gain/1 -> Mux/2
  Reshape/1 -> A_NL/1

== system Group69_Simulink/Relative Attitude/moving to LVLH and inertial/Subsystem ==
  r : Inport
  h_orb : Inport  Port=2
  Divide : Product  Inputs=*/
  Gain : Gain  Gain=[ 0 0 1]
  MATLAB Function : MATLAB Function  TreatAsAtomicUnit=on
  MATLAB Function1 : MATLAB Function  TreatAsAtomicUnit=on
  Square : Math  Operator=square  SaturateOnIntegerOverflow=on
  Terminator : Terminator
  Terminator2 : Terminator
  w_L : Outport
  wires:
  Gain/1 -> w_L/1
  r/1 -> MATLAB Function1/1(v)
  MATLAB Function/2(norm_v) -> Divide/1
  MATLAB Function1/1(v_hat) -> Terminator2/1
  Divide/1 -> Gain/1
  h_orb/1 -> MATLAB Function/1(v)
  MATLAB Function/1(v_hat) -> Terminator/1
  MATLAB Function1/2(norm_v) -> Square/1
  Square/1 -> Divide/2

== system Group69_Simulink/Sensors/Field of view check and r to body/If Action Subsystem ==
  v_hat : Inport
  Action Port : ActionPort  ActionPortLabel=if(u1> 90)
  Gain : Gain  Gain=0
  Out1 : Outport
  wires:
  Gain/1 -> Out1/1
  v_hat/1 -> Gain/1

== system Group69_Simulink/Sensors/Field of view check and r to body/If Action Subsystem1 ==
  v_hat : Inport
  Action Port : ActionPort  ActionPortLabel=else
  Out1 : Outport
  wires:
  v_hat/1 -> Out1/1

== system Group69_Simulink/Attitude Determination /A determination/Subsystem/If Action Subsystem ==
  In1 : Inport
  Action Port : ActionPort  ActionPortLabel=if(u1 == 2)
  Out1 : Outport
  wires:
  In1/1 -> Out1/1

== system Group69_Simulink/Attitude Determination /A determination/Subsystem/If Action Subsystem1 ==
  A : Inport
  Action Port : ActionPort  ActionPortLabel=else
  Out1 : Outport
  wires:
  A/1 -> Out1/1

== system Group69_Simulink/External torques/Magnetic Torque/mag_field in inertial/m_versor ==
  t : Inport
  Constant : Constant  Value=orbit.w_earth
  Constant1 : Constant  Value=11.5
  Cos : Trigonometry  Operator=cos
  Cos1 : Trigonometry  Operator=cos
  Degrees to Radians : simulink_extras/Transformations/Degrees to Radians
  Mux : Mux  Inputs=3
  Product : Product
  Product1 : Product
  Product2 : Product
  Reshape : Reshape  OutputDimensionality=Column vector (2-D)
  Sin : Trigonometry
  Sin1 : Trigonometry
  m : Outport
  wires:
  Constant1/1 -> Degrees to Radians/1
  Constant/1 -> Product/2
  t/1 -> Product/1
  Product/1 -> Sin1/1, Cos1/1
  Cos1/1 -> Product1/2
  Degrees to Radians/1 -> Cos/1, Sin/1
  Sin/1 -> Product2/1, Product1/1
  Sin1/1 -> Product2/2
  Product2/1 -> Mux/2
  Cos/1 -> Mux/3
  Product1/1 -> Mux/1
  Mux/1 -> Reshape/1
  Reshape/1 -> m/1

== matlab function Group69_Simulink/Relative Attitude/moving to LVLH and inertial/DCM from L to N/MATLAB Function ==
  data: v input; v_hat output
function v_hat = direction(v)

norm_v = norm(v);
v_hat = v/norm_v;



end

== matlab function Group69_Simulink/Relative Attitude/moving to LVLH and inertial/DCM from L to N/MATLAB Function1 ==
  data: v input; v_hat output
function v_hat = direction(v)

norm_v = norm(v);
v_hat = v/norm_v;



end

== matlab function Group69_Simulink/Relative Attitude/moving to LVLH and inertial/Subsystem/MATLAB Function ==
  data: v input; v_hat output; norm_v output
function [v_hat,norm_v] = elements(v)

norm_v = norm(v);
v_hat = v/norm_v;



end

== matlab function Group69_Simulink/Relative Attitude/moving to LVLH and inertial/Subsystem/MATLAB Function1 ==
  data: v input; v_hat output; norm_v output
function [v_hat,norm_v] = elements(v)

norm_v = norm(v);
v_hat = v/norm_v;



end

== matlab function Group69_Simulink/Kinematics/Orthonormality Check/MATLAB Function ==
  data: A input; detA output
function detA = determinant(A)

detA = det(A);
end

== matlab function Group69_Simulink/Attitude Determination /A determination/A_det ==
  data: A output; c output; b_s_hat input; r_s_hat input; b_N_hat input; r_N_hat input; A_dot output; wb_sens input; A_prev input
 function [A,c,A_dot]  = adet(b_s_hat,r_s_hat,b_N_hat,r_N_hat,wb_sens,A_prev)
 %%%%%%%%%%%%%%%%%%%%%%%%%%%%%%%%%%%%%%%%%%%%%%%%%%%%%%%%%%%%%%%%%%%%%%%%%%%%%%%%%%%%%%%
%
% adet: function useful to estimate the attitude determination by algebraic
%       method or by exploting gyroscope data (non-nominal condition)
%
% INPUTS:
%
% b_s_hat     [1x1]    Direction of the magnetic field vector by
%                      magnetic sensor
% r_s_hat     [1x1]    Direction of the position vector by horizon sensor
% b_N_hat     [1x1]    Direction of the magnetic field vector by
%                      Earth magnetic field model
% r_N_hat     [1x1]    Direction of the position vector by orbit
%                      propagation
% wb_sens     [3x1]    Angular velocities as output of the gyroscope 
% A_prev      [3x3]    DCM in non-nominal condition

%
% OUTPUTS:
%
% A           [3x3]    Observed DCM
% c           [1]      Distinction parameter (between nominal and
%                      non-nominal): -1 nominal, 2 non-nominal
% A_dot       [3x3]    Observed DCM derivative
%
% First Edition: 01/07/2023
%
% Authors: Rocco Larocca, Matteo Mascelloni, Davide Lanza, Afaq Shakeel
 
if  r_s_hat ~= zeros(3,1)
    
    % Nominal condition: both horizon and magnetic sensors are working, the
    % algebraic method can be applied

    s1 = r_s_hat;
    s2 = cross(r_s_hat,b_s_hat)/norm(cross(r_s_hat,b_s_hat));
    s3 = cross(s1,s2);
    v1 = r_N_hat;
    v2 = cross(r_N_hat,b_N_hat)/norm(cross(r_N_hat,b_N_hat));
    v3 = cross(v1,v2);
    S = [s1 s2 s3];
    V = [v1 v2 v3]; 
    A = S*V';
    A_dot = zeros(3);
    c =-1; 

else
   
    % Non-nominal condition: horizon sensor is not in FoV, magnetic sensor
    % can not produce an attitude determination alone. The gyroscope is
    % used to roughly estimate the DCM

    w_skew = [0 -wb_sens(3) wb_sens(2); wb_sens(3) 0 -wb_sens(1);-wb_sens(2) wb_sens(1) 0];
    A_dot = -w_skew*A_prev; 
    c = 2;
    A = zeros(3);


end

end

== matlab function Group69_Simulink/Attitude Determination /Orthonormality Check/MATLAB Function ==
  data: A input; detA output
function detA = determinant(A)

detA = det(A);
end

== matlab function Group69_Simulink/Attitude Determination /MATLAB Function ==
  data: v input; v_hat output
function v_hat = direction(v)



norm_v = norm(v);
v_hat = v/norm_v;



end

== matlab function Group69_Simulink/Attitude Determination /MATLAB Function1 ==
  data: v input; v_hat output
function v_hat = direction(v)

norm_v = norm(v);
v_hat = v/norm_v;



end

== matlab function Group69_Simulink/Attitude Determination /MATLAB Function2 ==
  data: v input; v_hat output
function v_hat = direction(v)

norm_v = norm(v);
v_hat = v/norm_v;



end

== matlab function Group69_Simulink/Sensors/Field of view check and r to body/MATLAB Function ==
  data: v input; v_hat output
function v_hat = direction(v)

norm_v = norm(v);
v_hat = v/norm_v;



end

== matlab function Group69_Simulink/External torques/Magnetic Torque/mag_field in inertial/MATLAB Function ==
  data: v input; v_hat output; norm_v output
function [v_hat,norm_v] = elements(v)

norm_v = norm(v);
v_hat = v/norm_v;



end

== matlab function Group69_Simulink/External torques/Gravity Gradient Torque/MATLAB Function ==
  data: v input; v_hat output; norm_v output
function [v_hat,norm_v] = elements(v)

norm_v = norm(v);
v_hat = v/norm_v;



end

== matlab function Group69_Simulink/Orbit/MATLAB Function ==
  data: v input; v_hat output; norm_v output
function [v_hat,norm_v] = elements(v)

norm_v = norm(v);
v_hat = v/norm_v;



end
